simulink model "flat_fading_and_diversity"  (Simulink 5.0)
settings: Solver=ode45  StartTime=0.0  StopTime=1000000.0  RelTol=1e-3
libraries: commdigbbndpm2 x4, commchan2 x3, commnoisgen2 x3, commsink2 x2, commrandsrc2 x2
settings Model: LastModifiedBy=Daiming Qu

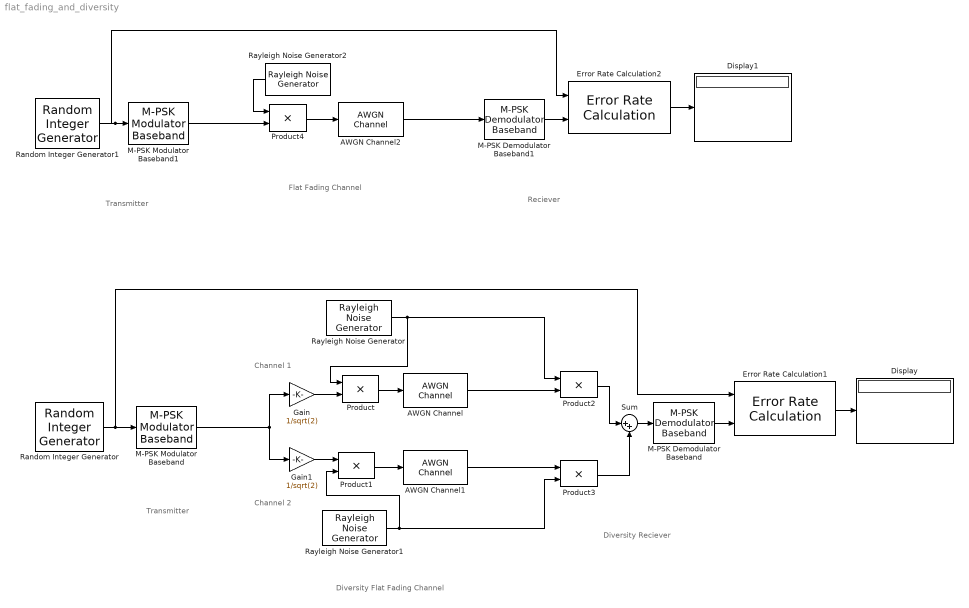
== system flat_fading_and_diversity ==
  note: Transmitter
  note: Diversity Reciever
  note: Transmitter
  note: Flat Fading Channel
  note: Diversity Flat Fading Channel
  note: Reciever
  note: Channel 1
  note: Channel 2
  AWGN Channel : commchan2/AWGN Channel  seed=67  noiseMode="Signal to noise ratio  (Es/No)"  EsNodB=20  SNRdB=20+3  Ps=1  Tsym=1  variance=1
  AWGN Channel1 : commchan2/AWGN Channel  seed=123  noiseMode="Signal to noise ratio  (Es/No)"  EsNodB=20  SNRdB=20+3  Ps=1  Tsym=1  variance=1
  AWGN Channel2 : commchan2/AWGN Channel  seed=67  noiseMode="Signal to noise ratio  (Es/No)"  EsNodB=20  SNRdB=20+3  Ps=1  Tsym=1  variance=1
  Display : Display
  Display1 : Display
  Error Rate Calculation1 : commsink2/Error Rate Calculation  N=0  st_delay=0  cp_mode=Entire frame  subframe=[]  PMode=Port  WsName=ErrorVec  RsMode2=off  stop=off  numErr=1000  maxBits=2e7
  Error Rate Calculation2 : commsink2/Error Rate Calculation  N=0  st_delay=0  cp_mode=Entire frame  subframe=[]  PMode=Port  WsName=ErrorVec  RsMode2=off  stop=off  numErr=1000  maxBits=2e7
  Gain : Gain  Gain=1/sqrt(2)  SaturateOnIntegerOverflow=on
  Gain1 : Gain  Gain=1/sqrt(2)  SaturateOnIntegerOverflow=on
  M-PSK Demodulator Baseband : commdigbbndpm2/M-PSK Demodulator Baseband  M=2  OutType=Integer  Dec=Binary  Ph=pi/4  numSamp=1
  M-PSK Demodulator Baseband1 : commdigbbndpm2/M-PSK Demodulator Baseband  M=2  OutType=Integer  Dec=Binary  Ph=pi/4  numSamp=1
  M-PSK Modulator Baseband : commdigbbndpm2/M-PSK Modulator Baseband  M=2  InType=Integer  Enc=Binary  Ph=pi/4  numSamp=1
  M-PSK Modulator Baseband1 : commdigbbndpm2/M-PSK Modulator Baseband  M=2  InType=Integer  Enc=Binary  Ph=pi/4  numSamp=1
  Product{,1..4} (5 alike) : Product  SaturateOnIntegerOverflow=on
  Random Integer Generator : commrandsrc2/Random Integer Generator  mul=2  seed=42  Ts=1  frameBased=off  sampPerFrame=128  orient=off
  Random Integer Generator1 : commrandsrc2/Random Integer Generator  mul=2  seed=386  Ts=1  frameBased=off  sampPerFrame=128  orient=off
  Rayleigh Noise Generator : commnoisgen2/Rayleigh Noise Generator  alpha=1/sqrt(2)  seed=345  Ts=1  frameBased=off  sampPerFrame=1  orient=off
  Rayleigh Noise Generator1 : commnoisgen2/Rayleigh Noise Generator  alpha=1/sqrt(2)  seed=75  Ts=1  frameBased=off  sampPerFrame=1  orient=off
  Rayleigh Noise Generator2 : commnoisgen2/Rayleigh Noise Generator  Orientation=left  alpha=1/sqrt(2)  seed=147  Ts=1  frameBased=off  sampPerFrame=1  orient=off
  Sum : Sum  Inputs=|++  SaturateOnIntegerOverflow=on
  wires:
  Product/1 -> AWGN Channel/1
  Error Rate Calculation1/1 -> Display/1
  Product1/1 -> AWGN Channel1/1
  AWGN Channel/1 -> Product2/2
  AWGN Channel1/1 -> Product3/1
  Product3/1 -> Sum/2
  M-PSK Modulator Baseband/1 -> Gain/1, Gain1/1
  Gain/1 -> Product/2
  Gain1/1 -> Product1/1
  Rayleigh Noise Generator1/1 -> Product3/2, Product1/2
  Rayleigh Noise Generator/1 -> Product2/1, Product/1
  M-PSK Demodulator Baseband/1 -> Error Rate Calculation1/2
  Product2/1 -> Sum/1
  Sum/1 -> M-PSK Demodulator Baseband/1
  Random Integer Generator/1 -> M-PSK Modulator Baseband/1, Error Rate Calculation1/1
  Product4/1 -> AWGN Channel2/1
  M-PSK Demodulator Baseband1/1 -> Error Rate Calculation2/2
  Error Rate Calculation2/1 -> Display1/1
  M-PSK Modulator Baseband1/1 -> Product4/2
  Rayleigh Noise Generator2/1 -> Product4/1
  AWGN Channel2/1 -> M-PSK Demodulator Baseband1/1
  Random Integer Generator1/1 -> Error Rate Calculation2/1, M-PSK Modulator Baseband1/1
